simulink model "mux21"  (R2024a)
settings: Solver=VariableStepAuto  StartTime=0.0  StopTime=10.0  RelTol=1e-3
settings Model: Creator=tusha  LastModifiedBy=tusha

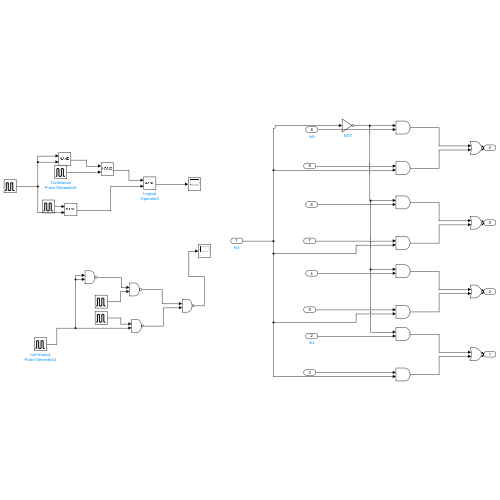
[thumbnail: Simulink's stored preview of the top-level diagram]
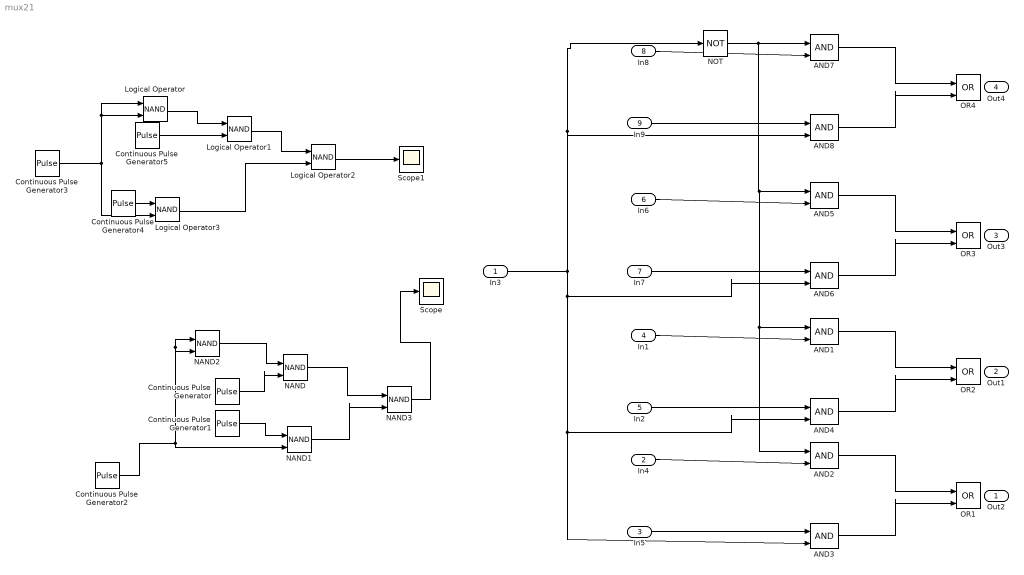
== system mux21 ==
  In3 : Inport
  In4 : Inport  Port=2
  In5 : Inport  Port=3
  In1 : Inport  Port=4
  In2 : Inport  Port=5
  In6 : Inport  Port=6
  In7 : Inport  Port=7
  In8 : Inport  Port=8
  In9 : Inport  Port=9
  AND{1..8} (8 alike) : Logic  IconShape=distinctive  AllPortsSameDT=off  OutDataTypeStr=boolean
  Continuous Pulse Generator{,1..5} (6 alike) : DiscretePulseGenerator  PulseType=Time based  Period=1  PulseWidth=50
  Logical Operator{,1..3} (4 alike) : Logic  Operator=NAND  AllPortsSameDT=off  OutDataTypeStr=boolean
  NAND{,1..3} (4 alike) : Logic  Operator=NAND  IconShape=distinctive  AllPortsSameDT=off  OutDataTypeStr=boolean
  NOT : Logic  Operator=NOT  IconShape=distinctive  AllPortsSameDT=off  OutDataTypeStr=boolean
  OR{1..4} (4 alike) : Logic  Operator=OR  IconShape=distinctive  AllPortsSameDT=off  OutDataTypeStr=boolean
  Scope : Scope
  Scope1 : Scope
  Out2 : Outport
  Out1 : Outport  Port=2
  Out3 : Outport  Port=3
  Out4 : Outport  Port=4
  wires:
  Continuous Pulse Generator2/1 -> NAND1/2, NAND2/2, NAND2/1
  NAND2/1 -> NAND/1
  Continuous Pulse Generator1/1 -> NAND1/1
  Continuous Pulse Generator/1 -> NAND/2
  NAND/1 -> NAND3/1
  NAND1/1 -> NAND3/2
  AND3/1 -> OR1/2
  AND2/1 -> OR1/1
  In4/1 -> AND2/2
  In5/1 -> AND3/1
  NAND3/1 -> Scope/1
  In2/1 -> AND4/1
  AND4/1 -> OR2/2
  In1/1 -> AND1/2
  AND1/1 -> OR2/1
  In7/1 -> AND6/1
  AND6/1 -> OR3/2
  In6/1 -> AND5/2
  AND5/1 -> OR3/1
  In9/1 -> AND8/1
  AND8/1 -> OR4/2
  In8/1 -> AND7/2
  AND7/1 -> OR4/1
  In3/1 -> AND6/2, AND4/2, AND3/2, NOT/1, AND8/2
  NOT/1 -> AND2/1, AND1/1, AND5/1, AND7/1
  Logical Operator3/1 -> Logical Operator2/2
  Continuous Pulse Generator5/1 -> Logical Operator1/2
  Continuous Pulse Generator3/1 -> Logical Operator/2, Logical Operator/1, Logical Operator3/2
  Continuous Pulse Generator4/1 -> Logical Operator3/1
  Logical Operator2/1 -> Scope1/1
  Logical Operator/1 -> Logical Operator1/1
  Logical Operator1/1 -> Logical Operator2/1
